simulink model "gain_test_uK"  (Simulink 8.4)
settings: Solver=ode45  StartTime=0.0  StopTime=10.0  RelTol=1e-3
settings Model: Creator=arnaud  LastModifiedBy=arnaud
settings DataIOCC: SaveFormat=Structure

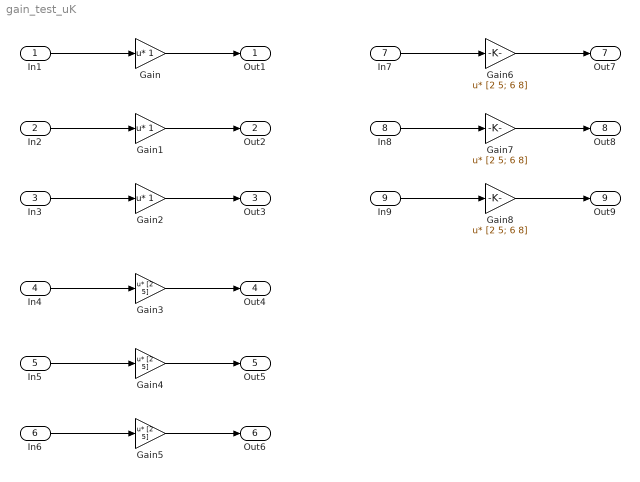
== system gain_test_uK ==
  In1 : Inport  OutDataTypeStr=double
  In2 : Inport  Port=2  OutDataTypeStr=int8
  In3 : Inport  Port=3  OutDataTypeStr=boolean
  In4 : Inport  Port=4  OutDataTypeStr=double
  In5 : Inport  Port=5  OutDataTypeStr=int8
  In6 : Inport  Port=6  OutDataTypeStr=boolean
  In7 : Inport  Port=7  OutDataTypeStr=double  PortDimensions=[2 2]
  In8 : Inport  Port=8  OutDataTypeStr=int8  PortDimensions=[2 2]
  In9 : Inport  Port=9  OutDataTypeStr=boolean  PortDimensions=[2 2]
  Gain : Gain  Multiplication=Matrix(u*K)
  Gain1 : Gain  Multiplication=Matrix(u*K)
  Gain2 : Gain  Multiplication=Matrix(u*K)
  Gain3 : Gain  Gain=[2 5]  Multiplication=Matrix(u*K)
  Gain4 : Gain  Gain=[2 5]  Multiplication=Matrix(u*K)
  Gain5 : Gain  Gain=[2 5]  Multiplication=Matrix(u*K)
  Gain6 : Gain  Gain=[2 5; 6 8]  Multiplication=Matrix(u*K)
  Gain7 : Gain  Gain=[2 5; 6 8]  Multiplication=Matrix(u*K)
  Gain8 : Gain  Gain=[2 5; 6 8]  Multiplication=Matrix(u*K)
  Out1 : Outport
  Out2 : Outport  Port=2
  Out3 : Outport  Port=3
  Out4 : Outport  Port=4
  Out5 : Outport  Port=5
  Out6 : Outport  Port=6
  Out7 : Outport  Port=7
  Out8 : Outport  Port=8
  Out9 : Outport  Port=9
  wires:
  In1/1 -> Gain/1
  Gain/1 -> Out1/1
  In2/1 -> Gain1/1
  Gain1/1 -> Out2/1
  In3/1 -> Gain2/1
  Gain2/1 -> Out3/1
  In4/1 -> Gain3/1
  Gain3/1 -> Out4/1
  In5/1 -> Gain4/1
  Gain4/1 -> Out5/1
  In6/1 -> Gain5/1
  Gain5/1 -> Out6/1
  In7/1 -> Gain6/1
  Gain6/1 -> Out7/1
  In8/1 -> Gain7/1
  Gain7/1 -> Out8/1
  In9/1 -> Gain8/1
  Gain8/1 -> Out9/1
